simulink model "Modeling_three_phase_inverter"  (R2023b)
settings: Solver=ode1  StartTime=0.0  StopTime=1.5  FixedStep=2e-6  RelTol=1e-3
InitFcn:
  | warning('off','physmod:simscape:engine:core:advancer_errors:fallback_solve')
libraries: nesl_utility x22, fl_lib x20, ee_lib x14, sdl_lib x1, eePwmGenerator x1
(part 3 of 3)

== matlab function Modeling_three_phase_inverter/MATLAB Function1 ==
  data: t input; halfCycleTime input; dutyCycle input; switchStates output
function switchStates = controlFullBridgeRectifier(t, halfCycleTime, dutyCycle)
    %controlFullBridgeRectifier(1, 0.5); % Simulate with 1 second half-cycle time and 50% duty cycle
    % Calculate the current cycle based on the global time
    currentCycle = floor(t / (2 * halfCycleTime)) + 1;

    % Calculate the time within the current half-cycle
    timeInHalfCycle = mod(t, 2 * halfCycleTime);

    % Determine the switch states based on the current half-cycle
    if timeInHalfCycle < halfCycleTime * dutyCycle
        %fprintf('Forward Direction at Time %.2f s (Cycle %d):\n', t, currentCycle);
        switchStates = [1, 0, 1, 0, 1, 0];  % Set the switches accordingly
    else
        %fprintf('Reverse Direction at Time %.2f s (Cycle %d):\n', t, currentCycle);
        switchStates = [0, 1, 0, 1, 0, 1];  % Set the switches accordingly
    end

    % Print and return the switch states
    printSwitchStates(switchStates);
end

function printSwitchStates(switchStates)
    fprintf('Switch States: ');
    disp(switchStates);
end
